simulink library "model_library"  (R2019b)
settings: Solver=VariableStepAuto  StartTime=0.0  StopTime=10.0  RelTol=1e-3
settings Model: Creator=Matt  LastModifiedBy=Watson
settings DataIOCC: ReturnWorkspaceOutputs=off
settings DebuggingCC: PregeneratedLibrarySubsystemCodeDiagnostic=none  ArithmeticOperatorsInVariantConditions=warning
settings SFSimCC: SimUseLocalCustomCode=off  CustomCodeUndefinedFunction=UseInterfaceOnly
settings RTWCC: RTWUseLocalCustomCode=off

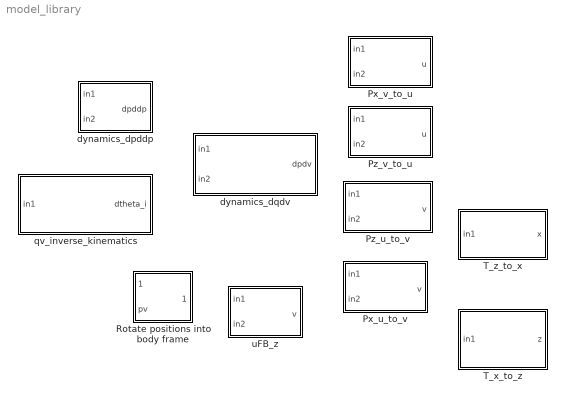
== system model_library ==
  Px_u_to_v : MATLAB Function  TreatAsAtomicUnit=on
  Px_v_to_u : MATLAB Function  TreatAsAtomicUnit=on
  Pz_u_to_v : MATLAB Function  TreatAsAtomicUnit=on
  Pz_v_to_u : MATLAB Function  TreatAsAtomicUnit=on
  Rotate positions into body frame : Subsystem
  T_x_to_z : MATLAB Function  TreatAsAtomicUnit=on
  T_z_to_x : MATLAB Function  TreatAsAtomicUnit=on
  dynamics_dpddp : MATLAB Function  TreatAsAtomicUnit=on
  dynamics_dqdv : MATLAB Function  TreatAsAtomicUnit=on
  qv_inverse_kinematics : MATLAB Function  TreatAsAtomicUnit=on
  uFB_z : MATLAB Function  TreatAsAtomicUnit=on

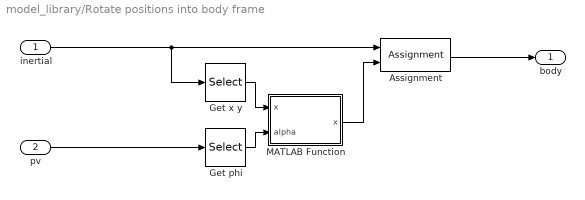
== system model_library/Rotate positions into body frame ==
  inertial : Inport
  pv : Inport  Port=2
  Assignment : Assignment  DiagnosticForDimensions=Warning  IndexOptions=Index vector (dialog)  Indices=1:2  OutputSizes=1
  Get phi : Selector  InputPortWidth=8  IndexOptions=Index vector (dialog)  Indices=3  OutputSizes=1
  Get x y : Selector  InputPortWidth=8  IndexOptions=Index vector (dialog)  Indices=1:2  OutputSizes=1
  MATLAB Function : MATLAB Function  TreatAsAtomicUnit=on
  body : Outport  VectorParamsAs1DForOutWhenUnconnected=off
  wires:
  inertial/1 -> Assignment/1, Get x y/1
  MATLAB Function/1(x) -> Assignment/2
  Get phi/1 -> MATLAB Function/2(alpha)
  Get x y/1 -> MATLAB Function/1("x ")
  Assignment/1 -> body/1
  pv/1 -> Get phi/1

== matlab function model_library/qv_inverse_kinematics ==
  data: in1 input; dtheta_i output
function dtheta_i = qv_inverse_kinematics(in1)
%#codegen

%    This function was generated by the Symbolic Math Toolbox version 8.4.
%    07-Jun-2020 11:42:38

stateInput5 = in1(5,:);
stateInput6 = in1(6,:);
stateInput7 = in1(7,:);
t2 = stateInput7.*(3.6e+1./1.7e+1);
t3 = stateInput7.*(6.0e+1./1.7e+1);
t4 = stateInput5.*3.361344537815126e+1;
t5 = stateInput6.*3.361344537815126e+1;
t6 = -t4;
t7 = -t5;
dtheta_i = [t3+t6+t7;t2+t4+t7;-t2+t6+t7;-t3+t4+t7];

== matlab function model_library/dynamics_dqdv ==
  data: in1 input; dpdv output; in2 input
function dpdv = dynamics_dqdv(in1,in2)
%#codegen

%    This function was generated by the Symbolic Math Toolbox version 8.4.
%    07-Jun-2020 11:42:38

stateInput3 = in1(3,:);
stateInput4 = in1(4,:);
stateInput5 = in1(5,:);
stateInput6 = in1(6,:);
stateInput7 = in1(7,:);
stateInput8 = in1(8,:);
tau_1 = in2(1,:);
tau_2 = in2(2,:);
tau_3 = in2(3,:);
tau_4 = in2(4,:);
t2 = cos(stateInput3);
t3 = cos(stateInput4);
t4 = sin(stateInput3);
t5 = sin(stateInput4);
t6 = stateInput4.*2.0;
t7 = stateInput7.^2;
t8 = stateInput8.^2;
t12 = tau_2.*(3.6e+1./1.7e+1);
t13 = tau_3.*(3.6e+1./1.7e+1);
t14 = tau_1.*(6.0e+1./1.7e+1);
t15 = tau_4.*(6.0e+1./1.7e+1);
t18 = stateInput5.*stateInput7.*(1.61e+2./5.0e+1);
t19 = stateInput6.*stateInput7.*(1.61e+2./5.0e+1);
t21 = tau_1.*3.361344537815126e+1;
t22 = tau_2.*3.361344537815126e+1;
t23 = tau_3.*3.361344537815126e+1;
t24 = tau_4.*3.361344537815126e+1;
t39 = stateInput8.*9.32e-5;
t40 = stateInput6.*3.132773109243698e-3;
t41 = stateInput8.*3.132773109243698e-3;
t43 = stateInput6.*9.956359014193912e-1;
t44 = stateInput7.*7.464282352941176e-3;
t45 = stateInput7.*2.090835392980722e-2;
t48 = stateInput5.*7.275862130948636e-2;
t49 = stateInput5.*6.493749673638682;
t9 = t3.^2;
t10 = sin(t6);
t11 = t5.^2;
t16 = -t13;
t17 = -t15;
t20 = -t19;
t25 = -t22;
t26 = -t24;
t27 = stateInput7.*stateInput8.*t3.*4.508e-1;
t28 = stateInput5.*stateInput7.*t3.*2.254e-1;
t29 = stateInput6.*stateInput7.*t5.*2.254e-1;
t30 = t5.*t7.*2.254e-1;
t31 = t5.*t8.*2.254e-1;
t33 = t5.*2.211174;
t46 = -t44;
t47 = -t45;
t51 = t5.*1.932700469060221e-9;
t53 = t5.*1.662431635466839e-14;
t32 = -t28;
t34 = -t33;
t35 = stateInput7.*stateInput8.*t10.*4.554437878787879e-2;
t37 = t7.*t10.*2.277218939393939e-2;
t42 = t9.*1.2086791428768e-11;
t50 = t5.*t9.*5.606471679904819e-10;
t54 = t5.*t9.*4.822462680186929e-15;
t56 = t9.*2.554188920360585e-13;
t58 = t11.*8.073674334265432e-13;
t59 = t9.*t11.*2.342050785026386e-13;
t63 = t20+t21+t23+t25+t26+t27+t47+t49;
t64 = t18+t21+t22+t23+t24+t30+t31+t41+t43;
t36 = -t35;
t38 = -t37;
t52 = -t50;
t55 = -t54;
t57 = -t56;
t60 = -t59;
t61 = t32+t34+t38+t39+t40+tau_1+tau_2+tau_3+tau_4;
t62 = t12+t14+t16+t17+t29+t36+t46+t48;
t65 = t42+t51+t52-4.166639697395127e-11;
t66 = t53+t55+t57+t58+t60+8.804971123180858e-13;
t67 = 1.0./(t53-t54+t57+t58+t60+8.804971123180858e-13);
dpdv = [stateInput5.*t2-stateInput6.*t4;stateInput6.*t2+stateInput5.*t4;stateInput7;stateInput8;t63.*t67.*(t9.*8.363203272615786e-11-t11.*3.905219265589605e-10+t9.*t11.*1.132845030404171e-10-2.883019448000656e-10).*8.850625e-4-t62.*t65.*t67.*8.850625e-4;-t61.*t67.*(t3.*1.133180532546843e-12+t3.*t5.*2.139513167784796e-14+t3.*t11.*1.039064234705584e-12)-t64.*t67.*(t5.*1.0724748384e-10+t11.*5.20852249933514e-9+5.680299737437486e-9).*4.491194675094697e-5;t62.*t67.*(t9.*8.584806753614885e-9-2.959412084247702e-8).*(-8.850625e-4)+t63.*t65.*t67.*8.850625e-4;t64.*t67.*(t3.*1.280339560818409e-9+t3.*t5.*2.4173582857536e-11+t3.*t11.*1.174000971350141e-9).*(-8.850625e-4)-t61.*t67.*(t5.*3.276090229454028e-13+t11.*1.591048018937218e-11+1.735161870832496e-11)];

== matlab function model_library/dynamics_dpddp ==
  data: in1 input; dpddp output; in2 input
function dpddp = dynamics_dpddp(in1,in2)
%#codegen

%    This function was generated by the Symbolic Math Toolbox version 8.1.
%    07-Mar-2019 13:59:27

stateInput3 = in1(3,:);
stateInput4 = in1(4,:);
stateInput5 = in1(5,:);
stateInput6 = in1(6,:);
stateInput7 = in1(7,:);
stateInput8 = in1(8,:);
tau_1 = in2(1,:);
tau_2 = in2(2,:);
tau_3 = in2(3,:);
tau_4 = in2(4,:);
t2 = sin(stateInput4);
t3 = cos(stateInput4);
t4 = t2.^2;
t5 = cos(stateInput3);
t6 = sin(stateInput3);
t7 = t4.*4.572209986109649e23;
t8 = t7+1.288212943991932e24;
t9 = 1.0./t8;
t10 = t2.*4.186608167497704e41;
t11 = t4.*2.41626622706705e42;
t12 = t10+t11+2.296250509914264e43;
t13 = 1.0./t12;
t14 = t6.^2;
t15 = t4.^2;
t16 = stateInput7.^2;
t17 = t15.*3.716462961258809e47;
t18 = t5.*tau_2.*(1.0e2./3.0);
t19 = t5.*tau_4.*(1.0e2./3.0);
t20 = t6.*tau_1.*(1.0e2./3.0);
t21 = t6.*tau_2.*(1.0e2./3.0);
t22 = t6.*tau_3.*(1.0e2./3.0);
t23 = t6.*tau_4.*(1.0e2./3.0);
t24 = stateInput8.^2;
t25 = t2.*(-1.9211904)+tau_1+tau_2+tau_3+tau_4-t2.*t3.*t16.*1.410048e-2;
t26 = t2.*5.721251257375662e46;
t27 = t14.*8.214431003240979e47;
t28 = t2.*t14.*5.721251257375662e46;
t29 = t5.*tau_1.*(1.0e2./3.0);
t30 = t5.*tau_3.*(1.0e2./3.0);
t31 = t2.*t5.*t16.*1.9584e-1;
t32 = t2.*t5.*t24.*1.9584e-1;
t33 = stateInput7.*stateInput8.*t3.*t6.*3.9168e-1;
t34 = t18+t19+t20-t21+t22-t23+t29+t30+t31+t32+t33-stateInput5.*stateInput7.*2.450711111111111e-1;
t35 = t2.*3.386822211933074e22;
t36 = t35-8.900254255973661e20;
t37 = tau_3.*(2.1e1./1.0e1);
t38 = tau_4.*(7.0./2.0);
t39 = stateInput5.*stateInput7.*t6.*5.146493333333333e-3;
t40 = stateInput4.*2.0;
t41 = sin(t40);
t42 = stateInput7.*stateInput8.*t41.*1.410048e-2;
t43 = t37+t38+t39+t42-tau_1.*(7.0./2.0)-tau_2.*(2.1e1./1.0e1)-stateInput6.*stateInput7.*t5.*5.146493333333333e-3;
t44 = t4.*1.539105139626841e48;
t45 = t2.*t6.*t16.*1.9584e-1;
t46 = t2.*t6.*t24.*1.9584e-1;
dpddp = [stateInput5;stateInput6;stateInput7;stateInput8;t3.*t6.*t9.*t25.*2.334666046828865e24+t5.*t13.*t36.*t43.*1.200959900632132e21+t9.*t13.*(t4.*1.869302417152916e48+t17+t27+t28-t4.*t14.*1.539105139626841e48-t14.*t15.*3.716462961258809e47+2.316520996504338e48).*(t18+t19+t20+t21+t22+t23+t45+t46-stateInput6.*stateInput7.*2.450711111111111e-1-t5.*tau_1.*(1.0e2./3.0)-t5.*tau_3.*(1.0e2./3.0)-stateInput7.*stateInput8.*t3.*t5.*3.9168e-1).*3.602879701896397e18-t5.*t6.*t9.*t13.*t34.*(t17-t26+t44-8.214431003240979e47).*3.602879701896397e18;t3.*t5.*t9.*t25.*-2.334666046828865e24+t6.*t13.*t36.*t43.*1.200959900632132e21-t9.*t13.*t34.*(t4.*3.301972775260748e47+t26-t27-t28+t4.*t14.*1.539105139626841e48+t14.*t15.*3.716462961258809e47+3.137964096828436e48).*3.602879701896397e18+t5.*t6.*t9.*t13.*(t17-t26+t44-8.214431003240979e47).*(t18+t19+t20+t21+t22+t23-t29-t30+t45+t46-stateInput6.*stateInput7.*2.450711111111111e-1-stateInput7.*stateInput8.*t3.*t5.*3.9168e-1).*3.602879701896397e18;-(tau_1.*-2.287223215381039e46-tau_2.*1.423640401869527e46+tau_3.*1.423640401869527e46+tau_4.*2.287223215381039e46-t2.*tau_1.*1.220231300130553e46+t2.*tau_2.*1.220231300130553e46-t2.*tau_3.*1.220231300130553e46+t2.*tau_4.*1.220231300130553e46+stateInput5.*stateInput7.*t6.*3.174587994655887e43-stateInput6.*stateInput7.*t5.*3.174587994655887e43+stateInput7.*stateInput8.*t3.*3.767947350747933e42+stateInput7.*stateInput8.*t41.*2.174639604360345e43+stateInput5.*stateInput7.*t2.*t6.*8.971303216066508e43-stateInput6.*stateInput7.*t2.*t5.*8.971303216066508e43)./(t2.*3.767947350747933e42+t4.*2.174639604360345e43+2.066625458922837e44);(t2.*-1.380281437023691e27+tau_1.*7.18451142075086e26+tau_2.*7.18451142075086e26+tau_3.*7.18451142075086e26+tau_4.*7.18451142075086e26-t16.*t41.*1.178874491710252e24+t24.*t41.*3.886378488193202e24+t3.*tau_1.*1.322977426536357e27+t3.*tau_2.*1.322977426536357e27+t3.*tau_3.*1.322977426536357e27+t3.*tau_4.*1.322977426536357e27-stateInput5.*stateInput7.*t3.*t5.*9.726706436885501e24-stateInput6.*stateInput7.*t3.*t6.*9.726706436885501e24)./(t3.^2.*7.772756976386404e24-2.967237702424925e25)];

== matlab function model_library/T_x_to_z ==
  data: in1 input; z output
function z = T_x_to_z(in1)
%#codegen

%    This function was generated by the Symbolic Math Toolbox version 8.4.
%    07-Jun-2020 11:43:02

stateInput1 = in1(1,:);
stateInput2 = in1(2,:);
stateInput3 = in1(3,:);
stateInput4 = in1(4,:);
stateInput5 = in1(5,:);
stateInput6 = in1(6,:);
stateInput7 = in1(7,:);
stateInput8 = in1(8,:);
t2 = cos(stateInput4);
t3 = sin(stateInput4);
t4 = t2.^2;
t5 = t3.^2;
t6 = t3.*1.662431635466839e-14;
t7 = t3.*t4.*4.822462680186929e-15;
t9 = t4.*2.554188920360585e-13;
t11 = t5.*8.073674334265432e-13;
t12 = t4.*t5.*2.342050785026386e-13;
t8 = -t7;
t10 = -t9;
t13 = -t12;
t14 = t6+t8+t10+t11+t13+8.804971123180858e-13;
t15 = 1.0./(t6-t7+t10+t11+t13+8.804971123180858e-13);
z = [stateInput1;stateInput2;stateInput3;stateInput4;stateInput5;stateInput6+(stateInput8.*(t15.*(t2.*1.133180532546843e-12+t2.*t3.*2.139513167784796e-14+t2.*t5.*1.039064234705584e-12).*2.975e-2+t15.*(t3.*1.0724748384e-10+t5.*5.20852249933514e-9+5.680299737437486e-9).*4.491194675094697e-5).*(t4.*4.49657419225e-5-1.550089173138068e-4))./(t2.*1.994930875e-4+9.08773621875e-5);stateInput7;stateInput8];

== matlab function model_library/Rotate positions into body frame/MATLAB Function ==
  data: x input; x output; alpha input
function x = rot2(x, alpha)

R = [cos(alpha) sin(alpha); -sin(alpha) cos(alpha)];

x = R*x;

== matlab function model_library/T_z_to_x ==
  data: in1 input; x output
function x = T_z_to_x(in1)
%#codegen

%    This function was generated by the Symbolic Math Toolbox version 8.1.
%    13-Dec-2018 16:19:18

z1 = in1(1,:);
z2 = in1(2,:);
z3 = in1(3,:);
z4 = in1(4,:);
z5 = in1(5,:);
z6 = in1(6,:);
z7 = in1(7,:);
z8 = in1(8,:);
t2 = cos(z4);
x = [z1;z2;z3;z4;z5;z6+(z8.*(t2.*5.434e3+3.3029e4).*1.297036692682703e16)./(t2.*2.349365796012602e21+1.70953125444395e21);z7;z8];

== matlab function model_library/Px_u_to_v ==
  data: in1 input; v output; in2 input
function v = Px_u_to_v(in1,in2)
%#codegen

%    This function was generated by the Symbolic Math Toolbox version 8.1.
%    13-Dec-2018 16:19:59

stateInput4 = in1(4,:);
u1 = in2(1,:);
u2 = in2(2,:);
u3 = in2(3,:);
t2 = sin(stateInput4);
t3 = t2.^2;
t4 = t3.*3.687446319870962e43;
t5 = t4+6.148308109415508e44;
t6 = 1.0./t5;
t7 = cos(stateInput4);
v = [t6.*(u1.*1.865910598615965e44+t3.*u1.*4.469246674877675e43-t2.*u3.*8.125903045232137e44);t6.*(u3.*1.970955346045949e46-t2.*u1.*8.125903045232137e44);-(u2.*(t7.*9.39746318405041e25+6.838125017775799e25))./(t7.^2.*1.276645373553248e25-5.646410780302922e25)];

== matlab function model_library/Pz_u_to_v ==
  data: in1 input; v output; in2 input
function v = Pz_u_to_v(in1,in2)
%#codegen

%    This function was generated by the Symbolic Math Toolbox version 8.1.
%    13-Dec-2018 16:21:17

u1 = in2(1,:);
u2 = in2(2,:);
u3 = in2(3,:);
z4 = in1(4,:);
t2 = sin(z4);
t3 = t2.^2;
t4 = t3.*3.687446319870962e43;
t5 = t4+6.148308109415508e44;
t6 = 1.0./t5;
t7 = cos(z4);
v = [t6.*(u1.*1.865910598615965e44+t3.*u1.*4.469246674877675e43-t2.*u3.*8.125903045232137e44);t6.*(u3.*1.970955346045949e46-t2.*u1.*8.125903045232137e44);-(u2.*(t7.*9.39746318405041e25+6.838125017775799e25))./(t7.^2.*1.276645373553248e25-5.646410780302922e25)];

== matlab function model_library/Px_v_to_u ==
  data: in1 input; u output; in2 input
function u = Px_v_to_u(in1,in2)
%#codegen

%    This function was generated by the Symbolic Math Toolbox version 8.1.
%    12-Dec-2018 11:40:28

stateInput4 = in1(4,:);
vin1 = in2(1,:);
vin2 = in2(2,:);
vin3 = in2(3,:);
t2 = cos(stateInput4);
t3 = sin(stateInput4);
u = [vin1.*3.295071111111111+t3.*vin3.*1.3585e-1;vin2.*(t2.^2.*1.276645373553248e25-5.646410780302922e25);t3.*vin1.*1.3585e-1+vin3.*(t3.^2.*7.47175e-3+3.119455812e-2)];

== matlab function model_library/Pz_v_to_u ==
  data: in1 input; u output; in2 input
function u = Pz_v_to_u(in1,in2)
%#codegen

%    This function was generated by the Symbolic Math Toolbox version 8.4.
%    07-Jun-2020 11:43:04

vin1 = in2(1,:);
vin2 = in2(2,:);
vin3 = in2(3,:);
z4 = in1(4,:);
t2 = cos(z4);
t3 = sin(z4);
t4 = t3.*2.254e-1;
t5 = t4-4.859317844784973e-3;
u = [vin1.*3.451396087846903+t5.*vin2;(vin3.*(t2.^2.*1.13056722548e+11-3.89736706389e+11).*(-1.06951871657754e-5))./(t2.*5.36452e+6+2.443761e+6);t5.*vin1+vin2.*(t3.^2.*4.554437878787879e-2+3.362303647058824e-2)];

== matlab function model_library/uFB_z ==
  data: in1 input; v output; in2 input
function v = uFB_z(in1,in2)
%#codegen

%    This function was generated by the Symbolic Math Toolbox version 8.4.
%    07-Jun-2020 11:43:01

w1 = in2(1,:);
w2 = in2(2,:);
w3 = in2(3,:);
z4 = in1(4,:);
z5 = in1(5,:);
z6 = in1(6,:);
z7 = in1(7,:);
z8 = in1(8,:);
t2 = cos(z4);
t3 = sin(z4);
t4 = z4.*2.0;
t5 = z7.^2;
t16 = z7.*7.464282352941176e-3;
t17 = z7.*2.090835392980722e-2;
t20 = z5.*7.275862130948636e-2;
t25 = z5.*6.493749673638682;
t6 = t2.^2;
t7 = sin(t4);
t8 = t3.^2;
t9 = t2.*z7.*z8.*4.508e-1;
t12 = t2.*1.994930875e-4;
t14 = t3.*1.0724748384e-10;
t18 = -t16;
t19 = -t17;
t24 = t2.*t3.*2.139513167784796e-14;
t27 = t3.*1.932700469060221e-9;
t29 = t3.*1.662431635466839e-14;
t33 = t2.*1.133180532546843e-12;
t10 = t7.*z7.*z8.*4.554437878787879e-2;
t13 = t6.*4.49657419225e-5;
t15 = t6.*1.2086791428768e-11;
t21 = t8.*5.20852249933514e-9;
t22 = t12+9.08773621875e-5;
t26 = t3.*t6.*5.606471679904819e-10;
t30 = t3.*t6.*4.822462680186929e-15;
t34 = t2.*t8.*1.039064234705584e-12;
t35 = t6.*2.554188920360585e-13;
t37 = t8.*8.073674334265432e-13;
t38 = t6.*t8.*2.342050785026386e-13;
t11 = -t10;
t23 = 1.0./t22;
t28 = -t26;
t31 = -t30;
t32 = t13-1.550089173138068e-4;
t36 = -t35;
t39 = -t38;
t40 = t14+t21+5.680299737437486e-9;
t41 = t24+t33+t34;
t42 = t15+t27+t28-4.166639697395127e-11;
t43 = t29+t31+t36+t37+t39+8.804971123180858e-13;
t44 = 1.0./(t29-t30+t36+t37+t39+8.804971123180858e-13);
t45 = t40.*t44.*4.491194675094697e-5;
t46 = t41.*t44.*2.975e-2;
t47 = t45+t46;
t48 = t23.*t32.*t47.*z8;
t49 = -t48;
t51 = z7.*(t48-z6).*(-1.61e+2./5.0e+1);
t52 = z7.*(t48-z6).*(1.61e+2./5.0e+1);
t53 = t3.*z7.*(t48-z6).*(-2.254e-1);
t50 = t49+z6;
t54 = t9+t19+t25+t52;
t55 = t11+t18+t20+t53;
v = [w1-t44.*t54.*(t6.*8.363203272615786e-11-t8.*3.905219265589605e-10+t6.*t8.*1.132845030404171e-10-2.883019448000656e-10).*8.850625e-4-t42.*t44.*(t10+t16-t20+t3.*z7.*(t48-z6).*2.254e-1).*8.850625e-4;w2-t42.*t44.*t54.*8.850625e-4-t44.*(t6.*8.584806753614885e-9-2.959412084247702e-8).*(t10+t16-t20+t3.*z7.*(t48-z6).*2.254e-1).*8.850625e-4;w3-t44.*(t3.*3.276090229454028e-13+t8.*1.591048018937218e-11+1.735161870832496e-11).*(t3.*2.211174+t48.*3.132773109243698e-3-z6.*3.132773109243698e-3-z8.*9.32e-5+t5.*t7.*2.277218939393939e-2+t2.*z5.*z7.*2.254e-1)+t44.*(t2.*1.280339560818409e-9+t2.*t3.*2.4173582857536e-11+t2.*t8.*1.174000971350141e-9).*(t48.*(-9.956359014193912e-1)+z6.*9.956359014193912e-1+z8.*3.132773109243698e-3+t3.*t5.*2.254e-1+z5.*z7.*(1.61e+2./5.0e+1)+t3.*z8.^2.*2.254e-1).*8.850625e-4];
